simulink library "libResultScoper"  (R2020b)
settings: Solver=VariableStepAuto  StartTime=0.0  StopTime=10.0  RelTol=1e-3
undefined symbols (not defined in the file): ft, s
libraries: aerolibconvert2 x3
settings Model: Creator=caatay  LastModifiedBy=caatay

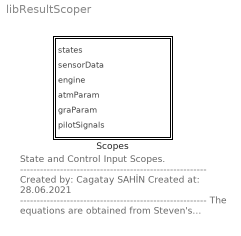
== system libResultScoper ==
  note: State and Control Input Scopes.
      | --------------------------------------------------------
      | Created by: Cagatay SAHİN
      | Created at: 28.06.2021
      | --------------------------------------------------------
      | The equations are obtained from
      | Steven's textbook.
      | The reference book can be found in
      | "references folder".
      | --------------------------------------------------------
      | for question:
      | cagataysahin44@gmail.com
  Scopes : Subsystem  mask(Flight Control System - Simulation Scopes){}
      mask help: Simulation Result grapher to obtain whole simulation results.
      mask Help:
      | This block integrate state derivative to state variables.
      | -------------------------------------------------------------------------------------------------------------------------------------------------
      | Inputs of this block set are:
      | 	states: Information of state variables.
      | 	sensorData: Information of sensor data.
      | 	engine: Information of engine.
      | 	atm: Information of atmosphere parameters.
      | 	gravity: Information of gravity Parameters.
      | 	commands: Information of pilot commands and flight surfaces
      | -------------------------------------------------------------------------------------------------------------------------------------------------
      | For question: "cagataysahin44@gmail.com"
      mask Display:
      | port_label('input',1,'Inf_{states}','texmode','on');
      | port_label('input',2,'Inf_{sensor}','texmode','on');
      | port_label('input',3,'Inf_{engine}','texmode','on');
      | port_label('input',4,'Inf_{atm}','texmode','on');
      | port_label('input',5,'Inf_{gravity}','texmode','on');
      | port_label('input',6,'Inf_{commands}','texmode','on');

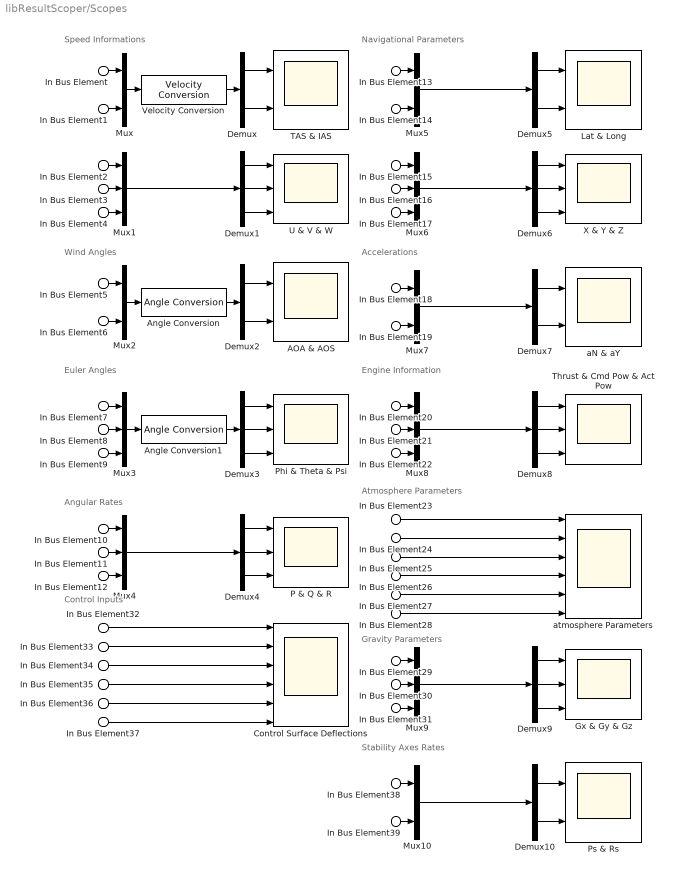
== system libResultScoper/Scopes ==
  note: Control Inputs
  note: Gravity Parameters
  note: Atmosphere Parameters
  note: Engine Information
  note: Accelerations
  note: Navigational Parameters
  note: Angular Rates
  note: Euler Angles
  note: Wind Angles
  note: Speed Informations
  note: Stability Axes Rates
  In Bus Element : Inport  PortName=states  Element=tas
  In Bus Element5 : Inport  PortName=states  Element=alpha
  In Bus Element6 : Inport  PortName=states  Element=beta
  In Bus Element7 : Inport  PortName=states  Element=phi
  In Bus Element8 : Inport  PortName=states  Element=theta
  In Bus Element9 : Inport  PortName=states  Element=psi
  In Bus Element10 : Inport  PortName=states  Element=p
  In Bus Element11 : Inport  PortName=states  Element=q
  In Bus Element12 : Inport  PortName=states  Element=r
  In Bus Element15 : Inport  PortName=states  Element=x_e
  In Bus Element16 : Inport  PortName=states  Element=y_e
  In Bus Element17 : Inport  PortName=states  Element=z_e
  In Bus Element22 : Inport  PortName=states  Element=power
  In Bus Element1 : Inport  Port=2  PortName=sensorData  Element=ias
  In Bus Element2 : Inport  Port=2  PortName=sensorData  Element=u
  In Bus Element3 : Inport  Port=2  PortName=sensorData  Element=v
  In Bus Element4 : Inport  Port=2  PortName=sensorData  Element=w
  In Bus Element14 : Inport  Port=2  PortName=sensorData  Element=long
  In Bus Element13 : Inport  Port=2  PortName=sensorData  Element=lat
  In Bus Element18 : Inport  Port=2  PortName=sensorData  Element=aN
  In Bus Element19 : Inport  Port=2  PortName=sensorData  Element=aY
  In Bus Element38 : Inport  Port=2  PortName=sensorData  Element=p_s
  In Bus Element39 : Inport  Port=2  PortName=sensorData  Element=r_s
  In Bus Element20 : Inport  Port=3  PortName=engine  Element=thrust
  In Bus Element21 : Inport  Port=3  PortName=engine  Element=cmdPow
  In Bus Element23 : Inport  Port=4  PortName=atmParam  Element=temp
  In Bus Element24 : Inport  Port=4  PortName=atmParam  Element=rho
  In Bus Element25 : Inport  Port=4  PortName=atmParam  Element=a
  In Bus Element26 : Inport  Port=4  PortName=atmParam  Element=mach
  In Bus Element27 : Inport  Port=4  PortName=atmParam  Element=qbar
  In Bus Element28 : Inport  Port=4  PortName=atmParam  Element=pSta
  In Bus Element29 : Inport  Port=5  PortName=graParam  Element=g_x
  In Bus Element31 : Inport  Port=5  PortName=graParam  Element=g_z
  In Bus Element30 : Inport  Port=5  PortName=graParam  Element=g_y
  In Bus Element32 : Inport  Port=6  PortName=pilotSignals  Element=thrtl
  In Bus Element33 : Inport  Port=6  PortName=pilotSignals  Element=ele
  In Bus Element34 : Inport  Port=6  PortName=pilotSignals  Element=ail
  In Bus Element35 : Inport  Port=6  PortName=pilotSignals  Element=rud
  In Bus Element36 : Inport  Port=6  PortName=pilotSignals  Element=sb
  In Bus Element37 : Inport  Port=6  PortName=pilotSignals  Element=lef
  AOA & AOS : Scope  NumInputPorts=2
  Angle Conversion : aerolibconvert2/Angle Conversion  IU=rad  OU=deg
  Angle Conversion1 : aerolibconvert2/Angle Conversion  IU=rad  OU=deg
  Control Surface Deflections : Scope  NumInputPorts=6
  Demux{,2,5,7,10} (5 alike) : Demux  Outputs=2
  Demux{1,3..4,6,8..9} (6 alike) : Demux  Outputs=3
  Gx & Gy & Gz : Scope  NumInputPorts=3
  Lat & Long : Scope  NumInputPorts=2
  Mux{,2,5,7,10} (5 alike) : Mux  Inputs=2
  Mux{1,3..4,6,8..9} (6 alike) : Mux  Inputs=3
  P & Q & R : Scope  NumInputPorts=3
  Phi & Theta & Psi : Scope  NumInputPorts=3
  Ps & Rs : Scope  NumInputPorts=2
  TAS & IAS : Scope  NumInputPorts=2
  Thrust & Cmd Pow & Act Pow : Scope  NumInputPorts=3
  U & V & W : Scope  NumInputPorts=3
  Velocity Conversion : aerolibconvert2/Velocity Conversion  IU=ft/s  OU=kts
  X & Y & Z : Scope  NumInputPorts=3
  aN & aY : Scope  NumInputPorts=2
  atmosphere Parameters : Scope  NumInputPorts=6
  wires:
  In Bus Element/1 -> Mux/1
  In Bus Element1/1 -> Mux/2
  Mux/1 -> Velocity Conversion/1
  Velocity Conversion/1 -> Demux/1
  Demux/2 -> TAS & IAS/2
  Demux/1 -> TAS & IAS/1
  In Bus Element2/1 -> Mux1/1
  In Bus Element3/1 -> Mux1/2
  In Bus Element4/1 -> Mux1/3
  Mux1/1 -> Demux1/1
  Demux1/3 -> U & V & W/3
  Demux1/2 -> U & V & W/2
  Demux1/1 -> U & V & W/1
  In Bus Element6/1 -> Mux2/2
  Mux2/1 -> Angle Conversion/1
  Demux2/2 -> AOA & AOS/2
  In Bus Element5/1 -> Mux2/1
  Demux2/1 -> AOA & AOS/1
  Angle Conversion/1 -> Demux2/1
  Mux3/1 -> Angle Conversion1/1
  In Bus Element7/1 -> Mux3/1
  Demux3/1 -> Phi & Theta & Psi/1
  Demux3/3 -> Phi & Theta & Psi/3
  In Bus Element9/1 -> Mux3/3
  Demux3/2 -> Phi & Theta & Psi/2
  In Bus Element8/1 -> Mux3/2
  Angle Conversion1/1 -> Demux3/1
  Mux4/1 -> Demux4/1
  In Bus Element11/1 -> Mux4/2
  Demux4/1 -> P & Q & R/1
  Demux4/3 -> P & Q & R/3
  In Bus Element12/1 -> Mux4/3
  In Bus Element10/1 -> Mux4/1
  Demux4/2 -> P & Q & R/2
  Demux5/1 -> Lat & Long/1
  Mux6/1 -> Demux6/1
  In Bus Element15/1 -> Mux6/1
  In Bus Element14/1 -> Mux5/2
  Mux5/1 -> Demux5/1
  In Bus Element13/1 -> Mux5/1
  Demux6/1 -> X & Y & Z/1
  Demux6/2 -> X & Y & Z/2
  In Bus Element16/1 -> Mux6/2
  Demux5/2 -> Lat & Long/2
  In Bus Element17/1 -> Mux6/3
  Demux6/3 -> X & Y & Z/3
  In Bus Element19/1 -> Mux7/2
  Demux7/1 -> aN & aY/1
  Demux7/2 -> aN & aY/2
  Mux7/1 -> Demux7/1
  In Bus Element18/1 -> Mux7/1
  Mux8/1 -> Demux8/1
  In Bus Element21/1 -> Mux8/2
  Demux8/1 -> Thrust & Cmd Pow & Act Pow/1
  Demux8/3 -> Thrust & Cmd Pow & Act Pow/3
  In Bus Element22/1 -> Mux8/3
  In Bus Element20/1 -> Mux8/1
  Demux8/2 -> Thrust & Cmd Pow & Act Pow/2
  In Bus Element28/1 -> atmosphere Parameters/6
  In Bus Element27/1 -> atmosphere Parameters/5
  In Bus Element26/1 -> atmosphere Parameters/4
  In Bus Element25/1 -> atmosphere Parameters/3
  In Bus Element24/1 -> atmosphere Parameters/2
  In Bus Element23/1 -> atmosphere Parameters/1
  Demux9/1 -> Gx & Gy & Gz/1
  In Bus Element30/1 -> Mux9/2
  Demux9/3 -> Gx & Gy & Gz/3
  Mux9/1 -> Demux9/1
  In Bus Element31/1 -> Mux9/3
  In Bus Element29/1 -> Mux9/1
  Demux9/2 -> Gx & Gy & Gz/2
  In Bus Element37/1 -> Control Surface Deflections/6
  In Bus Element36/1 -> Control Surface Deflections/5
  In Bus Element35/1 -> Control Surface Deflections/4
  In Bus Element34/1 -> Control Surface Deflections/3
  In Bus Element33/1 -> Control Surface Deflections/2
  In Bus Element32/1 -> Control Surface Deflections/1
  In Bus Element38/1 -> Mux10/1
  Demux10/1 -> Ps & Rs/1
  Mux10/1 -> Demux10/1
  Demux10/2 -> Ps & Rs/2
  In Bus Element39/1 -> Mux10/2
